simulink model "lab6"  (R2021a)
settings: Solver=VariableStepAuto  StartTime=0.0  StopTime=20.0  RelTol=1e-3
libraries: simulink x9
settings Model: Creator=vedve  LastModifiedBy=vedve

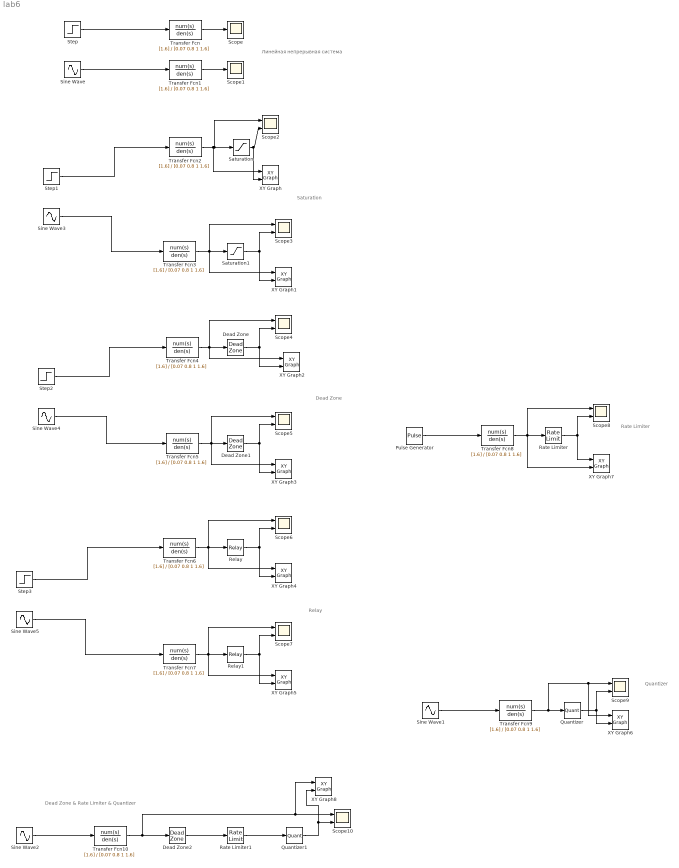
== system lab6 ==
  note: Линейная непрерывная система
  note: Saturation
  note: Dead Zone
  note: Relay
  note: Quantizer
  note: Rate Limiter
  note: Dead Zone & Rate Limiter & Quantizer
  Dead Zone : DeadZone  LowerValue=0.9  UpperValue=1.1  SaturateOnIntegerOverflow=on
  Dead Zone1 : DeadZone  LowerValue=0.9  UpperValue=1.1  SaturateOnIntegerOverflow=on
  Dead Zone2 : DeadZone  LowerValue=0.9  UpperValue=1.1  SaturateOnIntegerOverflow=on
  Pulse Generator : DiscretePulseGenerator  PulseType=Time based  Period=6  PulseWidth=50
  Quantizer : Quantizer
  Quantizer1 : Quantizer
  Rate Limiter : RateLimiter  RisingSlewLimit=0.5  FallingSlewLimit=-0.5  SampleTimeMode=inherited
  Rate Limiter1 : RateLimiter  RisingSlewLimit=0.5  FallingSlewLimit=-0.5  SampleTimeMode=inherited
  Relay : Relay  OnSwitchValue=1.1  OffSwitchValue=0.9  OnOutputValue=1.5  OffOutputValue=-0.5
  Relay1 : Relay  OnSwitchValue=1.1  OffSwitchValue=0.9  OnOutputValue=1.5  OffOutputValue=-0.5
  Saturation : Saturate  UpperLimit=1.1  LowerLimit=0.9
  Saturation1 : Saturate  UpperLimit=1.1  LowerLimit=0.9
  Scope : Scope
  Scope1 : Scope
  Scope{2..10} (9 alike) : Scope  NumInputPorts=2
  Sine Wave{,3..5} (4 alike) : Sin  Amplitude=2  SampleTime=0
  Sine Wave1 : Sin  SampleTime=0
  Sine Wave2 : Sin  SampleTime=0
  Step{,1..3} (4 alike) : Step  SampleTime=0
  Transfer Fcn{,1..10} (11 alike) : TransferFcn  Numerator=[1.6]  Denominator=[0.07 0.8 1 1.6]
  XY Graph : simulink/Sinks/XY Graph  xmin=-1  xmax=2  ymin=-1  ymax=2  st=-1
  XY Graph1 : simulink/Sinks/XY Graph  xmin=-2  xmax=2  ymin=-2  ymax=2  st=-1
  XY Graph2 : simulink/Sinks/XY Graph  xmin=-2  xmax=2  ymin=-2  ymax=2  st=-1
  XY Graph{3..6,8} (5 alike) : simulink/Sinks/XY Graph  xmin=-2  xmax=2  ymin=-4  ymax=2  st=-1
  XY Graph7 : simulink/Sinks/XY Graph  xmin=-2  xmax=2  ymin=-2  ymax=2  st=-1
  wires:
  Transfer Fcn/1 -> Scope/1
  Transfer Fcn1/1 -> Scope1/1
  Transfer Fcn2/1 -> XY Graph/1, Scope2/1, Saturation/1
  Saturation/1 -> XY Graph/2, Scope2/2
  Saturation1/1 -> XY Graph1/2, Scope3/2
  Transfer Fcn3/1 -> XY Graph1/1, Scope3/1, Saturation1/1
  Transfer Fcn4/1 -> XY Graph2/1, Scope4/1, Dead Zone/1
  Dead Zone/1 -> XY Graph2/2, Scope4/2
  Dead Zone1/1 -> Scope5/2, XY Graph3/2
  Transfer Fcn5/1 -> Scope5/1, XY Graph3/1, Dead Zone1/1
  Transfer Fcn6/1 -> XY Graph4/1, Scope6/1, Relay/1
  Relay/1 -> XY Graph4/2, Scope6/2
  Relay1/1 -> Scope7/2, XY Graph5/2
  Transfer Fcn7/1 -> Relay1/1, Scope7/1, XY Graph5/1
  Rate Limiter/1 -> XY Graph7/1, Scope8/2
  Pulse Generator/1 -> Transfer Fcn8/1
  Transfer Fcn8/1 -> XY Graph7/2, Rate Limiter/1, Scope8/1
  Transfer Fcn9/1 -> XY Graph6/1, Scope9/1, Quantizer/1
  Sine Wave1/1 -> Transfer Fcn9/1
  Quantizer/1 -> XY Graph6/2, Scope9/2
  Sine Wave2/1 -> Transfer Fcn10/1
  Transfer Fcn10/1 -> Dead Zone2/1, XY Graph8/1, Scope10/1
  Dead Zone2/1 -> Rate Limiter1/1
  Rate Limiter1/1 -> Quantizer1/1
  Quantizer1/1 -> XY Graph8/2, Scope10/2
  Step/1 -> Transfer Fcn/1
  Sine Wave/1 -> Transfer Fcn1/1
  Sine Wave3/1 -> Transfer Fcn3/1
  Step1/1 -> Transfer Fcn2/1
  Step2/1 -> Transfer Fcn4/1
  Sine Wave4/1 -> Transfer Fcn5/1
  Sine Wave5/1 -> Transfer Fcn7/1
  Step3/1 -> Transfer Fcn6/1
